simulink model "ukf_cfg2"  (R2013b)
settings: Solver=FixedStepDiscrete  StartTime=0.0  StopTime=400  FixedStep=0.02  RelTol=1e-3
undefined symbols (not defined in the file): steering_ratio
libraries: simulink x2
settings Model: Creator=igeorgie  LastModifiedBy=igeorgie

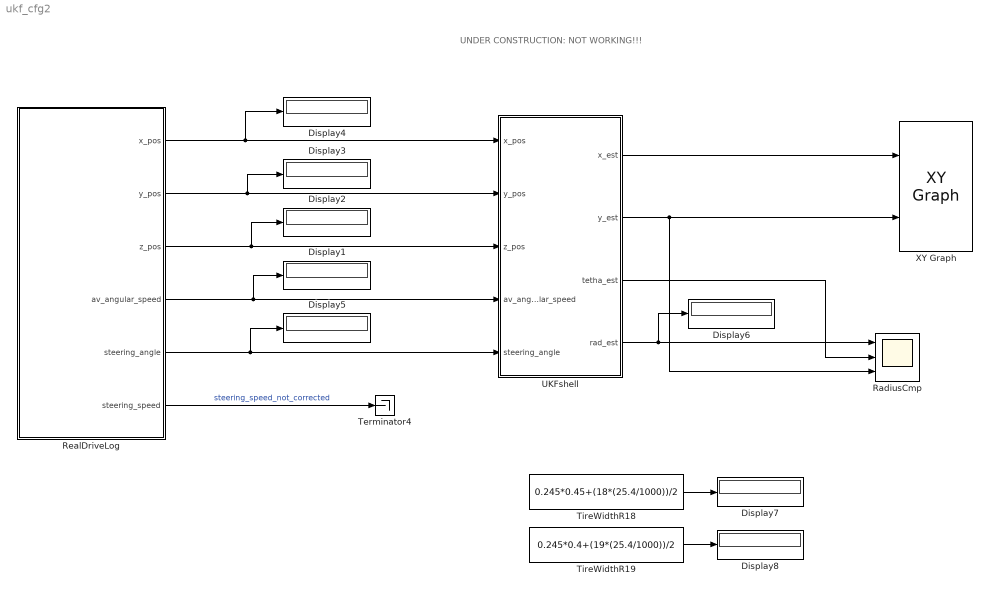
== system ukf_cfg2 ==
  note: UNDER CONSTRUCTION: NOT WORKING!!!
  Display{1..8} (8 alike) : Display
  RadiusCmp : Scope  NumInputPorts=3
      settings: YMin=-5~-5~-5  YMax=5~5~5  MaxDataPoints=50000
  RealDriveLog : Subsystem
  Terminator4 : Terminator
  TireWidthR18 : Constant  Value=0.245*0.45+(18*(25.4/1000))/2
  TireWidthR19 : Constant  Value=0.245*0.4+(19*(25.4/1000))/2
  UKFshell : Subsystem
  XY Graph : simulink/Sinks/XY Graph  xmin=0  xmax=1000  ymin=0  ymax=1000  st=0.02
  wires:
  RealDriveLog/6(steering_speed) -> Terminator4/1  "steering_speed_not_corrected"
  RealDriveLog/1(x_pos) -> Display4/1, UKFshell/1(x_pos)
  RealDriveLog/3(z_pos) -> Display2/1, UKFshell/3(z_pos)
  UKFshell/3(tetha_est) -> RadiusCmp/2
  RealDriveLog/4(av_angular_speed) -> Display1/1, UKFshell/4(av_angular_speed)
  RealDriveLog/2(y_pos) -> Display3/1, UKFshell/2(y_pos)
  UKFshell/4(rad_est) -> RadiusCmp/1, Display6/1
  RealDriveLog/5(steering_angle) -> Display5/1, UKFshell/5(steering_angle)
  UKFshell/1(x_est) -> XY Graph/1
  UKFshell/2(y_est) -> RadiusCmp/3, XY Graph/2
  TireWidthR18/1 -> Display7/1
  TireWidthR19/1 -> Display8/1

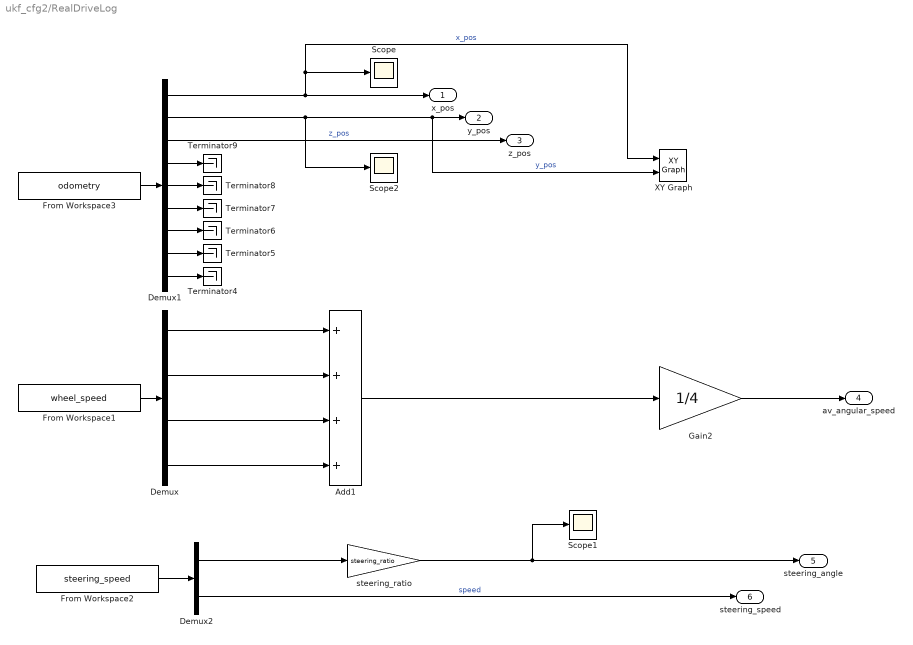
== system ukf_cfg2/RealDriveLog ==
  Add1 : Sum  Inputs=++++
  Demux : Demux
  Demux1 : Demux  Outputs=9
  Demux2 : Demux  Outputs=2
  From Workspace1 : FromWorkspace  VariableName=wheel_speed  SampleTime=0.02  Interpolate=off  OutputAfterFinalValue=Holding final value
  From Workspace2 : FromWorkspace  VariableName=steering_speed  SampleTime=0.02  Interpolate=off  OutputAfterFinalValue=Holding final value
  From Workspace3 : FromWorkspace  VariableName=odometry  Interpolate=off  OutputAfterFinalValue=Holding final value
  Gain2 : Gain  Gain=1/4
  Scope : Scope
      settings: YMin=132850  YMax=133375  SaveName=ScopeData2
  Scope1 : Scope
      settings: SaveName=ScopeData4
  Scope2 : Scope
      settings: SaveName=ScopeData5
  Terminator{4..9} (6 alike) : Terminator
  XY Graph : simulink/Sinks/XY Graph  xmin=0  xmax=1000  ymin=0  ymax=1000  st=0.02
  steering_ratio : Gain  Gain=steering_ratio
  x_pos : Outport
  y_pos : Outport  Port=2
  z_pos : Outport  Port=3
  av_angular_speed : Outport  Description=|  Port=4
      | w=(w3+w4)/2
      | Units [rad/sec]
      settings: AttributesFormatString=%<Description>
  steering_angle : Outport  Description=Units [rad]  Port=5
      settings: AttributesFormatString=%<Description>
  steering_speed : Outport  Description=Units [m/s]  Port=6
      settings: AttributesFormatString=%<Description>
  wires:
  Demux2/2 -> steering_speed/1  "speed"
  Demux/4 -> Add1/4
  Demux/2 -> Add1/2
  Demux/1 -> Add1/1
  Demux/3 -> Add1/3
  From Workspace1/1 -> Demux/1
  From Workspace2/1 -> Demux2/1
  Demux2/1 -> steering_ratio/1
  From Workspace3/1 -> Demux1/1
  Demux1/9 -> Terminator4/1
  Demux1/8 -> Terminator5/1
  Demux1/6 -> Terminator7/1
  Demux1/7 -> Terminator6/1
  Demux1/5 -> Terminator8/1
  Demux1/4 -> Terminator9/1
  Demux1/1 -> XY Graph/1, Scope/1, x_pos/1  "x_pos"
  Demux1/2 -> XY Graph/2, y_pos/1, Scope2/1  "y_pos"
  Demux1/3 -> z_pos/1  "z_pos"
  Add1/1 -> Gain2/1
  Gain2/1 -> av_angular_speed/1
  steering_ratio/1 -> Scope1/1, steering_angle/1

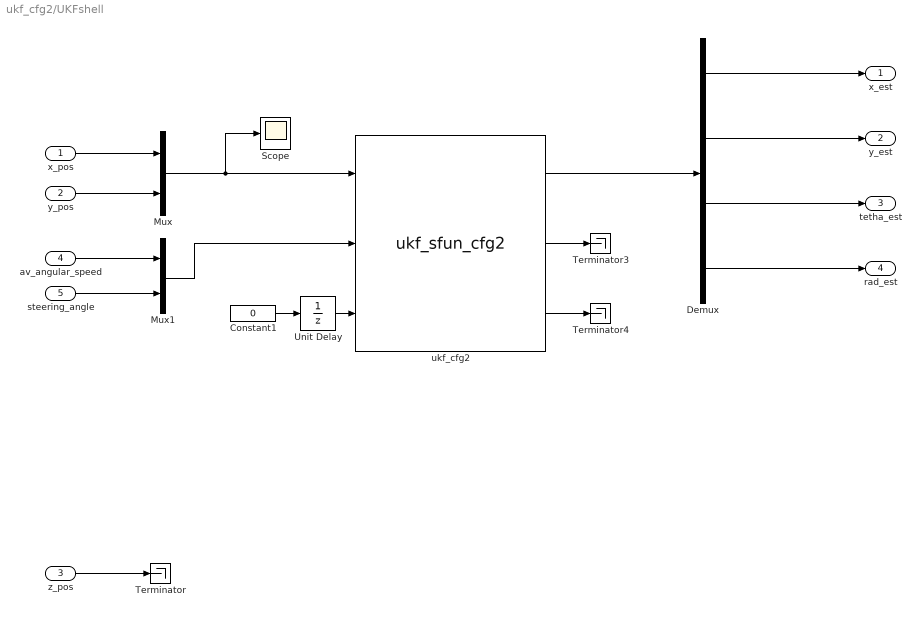
== system ukf_cfg2/UKFshell ==
  x_pos : Inport
  y_pos : Inport  Port=2
  z_pos : Inport  Port=3
  av_angular_speed : Inport  Port=4
  steering_angle : Inport  Port=5
  Constant1 : Constant  Value=0  OutDataTypeStr=double  SampleTime=0.02
  Demux : Demux
  Mux : Mux  Inputs=2
  Mux1 : Mux  Inputs=2
  Scope : Scope
  Terminator : Terminator
  Terminator3 : Terminator
  Terminator4 : Terminator
  Unit Delay : UnitDelay  InitialCondition=1  SampleTime=0.02
  ukf_cfg2 : S-Function  InitFcn=try, set_param(gcb,'FunctionName','ukf_sfun_cfg2'), end  FunctionName=ukf_sfun_cfg2  SFunctionModules=ukf_sfun_cfg2_wrapper ukfLib mtxLib ukfCfg2  EnableBusSupport=off  mask(S-Function Builder){}
      mask help: Simulink:masks:SFunctionBuilder_MD
      mask init:
      | val = [[.9  0.75 0.75 1 1 .9 .9 1]',[1 1 0.75 0.75 .9 .9 1 .9]'];try , sys = get_param(gcb,'SfunBuilderFcnName');if isempty(sys), sys = get_param(gcb,'FunctionName'); end,catch, sys = get_param(gcb,'FunctionName'); end
      settings: CopyFcn=set_param(gcbh,'LinkStatus','none')  PreSaveFcn=try, set_param(gcb,'FunctionName','ukf_sfun_cfg2'), end  OpenFcn=sfunctionwizard(gcbh)
      mask Display: plot(val(:,1),val(:,2)),disp(sys), port_label('input',1,'meas'), port_label('input',2,'input'), port_label('input',3,'Init'), port_label('output',1,'states'), port_label('output',2,'y_mean'), port_label('output',3,'kalman')
  x_est : Outport
  y_est : Outport  Port=2
  tetha_est : Outport  Port=3
  rad_est : Outport  Port=4
  wires:
  z_pos/1 -> Terminator/1
  y_pos/1 -> Mux/2
  x_pos/1 -> Mux/1
  Demux/1 -> x_est/1
  Demux/2 -> y_est/1
  Demux/4 -> rad_est/1
  ukf_cfg2/1 -> Demux/1
  Demux/3 -> tetha_est/1
  ukf_cfg2/2 -> Terminator3/1
  ukf_cfg2/3 -> Terminator4/1
  Constant1/1 -> Unit Delay/1
  Unit Delay/1 -> ukf_cfg2/3
  Mux/1 -> Scope/1, ukf_cfg2/1
  av_angular_speed/1 -> Mux1/1
  steering_angle/1 -> Mux1/2
  Mux1/1 -> ukf_cfg2/2
